simulink model "SEA_modelDEE"  (Simulink 8.1)
settings: Solver=ode45  StartTime=0.0  StopTime=10.0  RelTol=1e-3
values from neighbouring files (symbols this model uses):
  b = 0.0575    [TSC150918ProvaMatlab.m]
  d = 2.5185    [TSC150918ProvaMatlab.m]
  g = 9.81    [TSC150918ProvaMatlab.m]
  j = 0.2156    [TSC150918ProvaMatlab.m]
  k = 200    [TSC150918ProvaMatlab.m]
  l = 0.5    [TSC150918ProvaMatlab.m]
  m = 0.15    [TSC150918ProvaMatlab.m]
  X0 = Xe + Dx0    [TSC150918ProvaMatlab.m]
settings Model: Creator=lbiagiotti  LastModifiedBy=peppe
settings DebuggingCC: StrictBusMsg=Warning

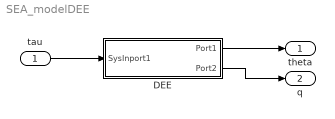
== system SEA_modelDEE ==
  tau : Inport
  DEE : Subsystem  mask(Differential Equation Editor (DEE)){}
      settings: OpenFcn=diffeqed
      mask Display: disp('Differential Equation\n Editor')
  theta : Outport
  q : Outport  Port=2
  wires:
  tau/1 -> DEE/1(SysInport1)
  DEE/1(Port1) -> theta/1
  DEE/2(Port2) -> q/1

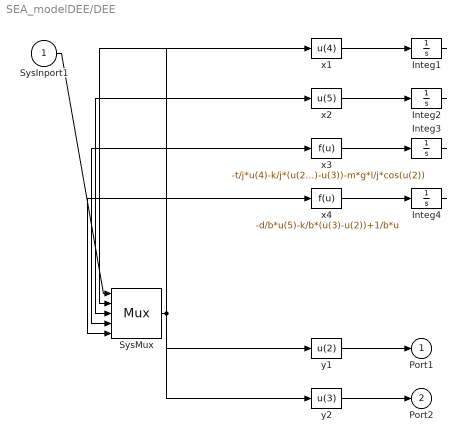
== system SEA_modelDEE/DEE ==
  SysInport1 : Inport
  Integ1 : Integrator  InitialCondition=X0(1)
  Integ2 : Integrator  InitialCondition=X0(2)
  Integ3 : Integrator  InitialCondition=X0(3)
  Integ4 : Integrator  InitialCondition=X0(4)
  SysMux : Mux  Inputs=5
  x1 : Fcn  Expr=u(4)
  x2 : Fcn  Expr=u(5)
  x3 : Fcn  Expr=-t/j*u(4)-k/j*(u(2)-u(3))-m*g*l/j*cos(u(2))
  x4 : Fcn  Expr=-d/b*u(5)-k/b*(u(3)-u(2))+1/b*u
  y1 : Fcn  Expr=u(2)
  y2 : Fcn  Expr=u(3)
  Port1 : Outport
  Port2 : Outport  Port=2
  wires:
  SysInport1/1 -> SysMux/1
  SysMux/1 -> x1/1, x2/1, x3/1, x4/1, y1/1, y2/1
  x1/1 -> Integ1/1
  Integ1/1 -> SysMux/2
  x2/1 -> Integ2/1
  Integ2/1 -> SysMux/3
  x3/1 -> Integ3/1
  Integ3/1 -> SysMux/4
  x4/1 -> Integ4/1
  Integ4/1 -> SysMux/5
  y1/1 -> Port1/1
  y2/1 -> Port2/1
